simulink model "Lab_3_exerciszcxe"  (R2018a)
settings: Solver=VariableStepAuto  StartTime=0.0  StopTime=7  RelTol=1e-3
libraries: powerlib_extras x7, simulink x3
settings Model: Creator=WIN  LastModifiedBy=WIN

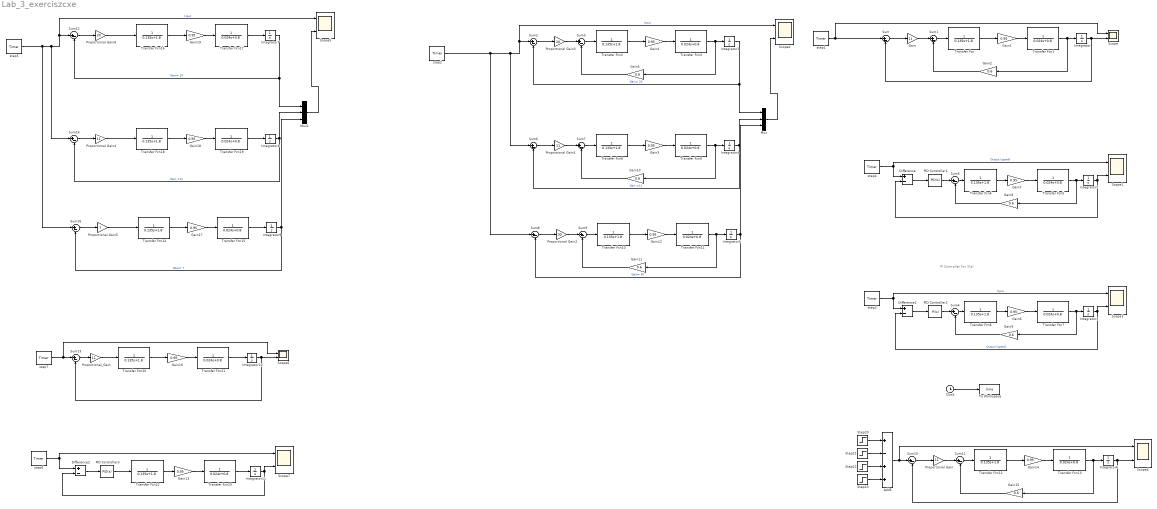
== system Lab_3_exerciszcxe ==
  note: PI Controller For 3(a)
  Add5 : Sum  Inputs=+-++
  Clock : Clock
  Difference : Sum  Inputs=+-
  Difference1 : Sum  Inputs=+-
  Difference2 : Sum  Inputs=+-
  Gain : Gain  Gain=11
  Gain{1,3..4,6..7,12..14,16..19} (12 alike) : Gain  Gain=0.95
  Gain{2,5,8..11,15} (7 alike) : Gain  Gain=0.6
  Integrator{,1..11} (12 alike) : Integrator
  Mux : Mux  Inputs=3
  Mux1 : Mux  Inputs=3
  PID Controller1 : simulink/Continuous/PID Controller  Controller=PID  TimeDomain=Continuous-time  SampleTime=-1  IntegratorMethod=Forward Euler  FilterMethod=Forward Euler  Form=Parallel  UseFilter=on  ControllerParametersSource=internal  P=26  I=12  D=1.5  N=100  InitialConditionSource=internal  InitialConditionForIntegrator=0  InitialConditionForFilter=0  ExternalReset=none  ZeroCross=off  LimitOutput=off  UpperSaturationLimit=inf  LowerSaturationLimit=-inf  LinearizeAsGain=on  AntiWindupMode=none  Kb=1  TrackingMode=off  Kt=1  PParamMin=[]  PParamMax=[]  IParamMin=[]  IParamMax=[]  DParamMin=[]  DParamMax=[]  NParamMin=[]  NParamMax=[]  KbParamMin=[]  KbParamMax=[]  KtParamMin=[]  KtParamMax=[]  POutMin=[]  POutMax=[]  IOutMin=[]  IOutMax=[]  DOutMin=[]  DOutMax=[]  NOutMin=[]  NOutMax=[]  KbOutMin=[]  KbOutMax=[]  KtOutMin=[]  KtOutMax=[]  IntegratorOutMin=[]  IntegratorOutMax=[]  FilterOutMin=[]  FilterOutMax=[]  SumOutMin=[]  SumOutMax=[]  SumI1OutMin=[]  SumI1OutMax=[]  SumI2OutMin=[]  SumI2OutMax=[]  SumI3OutMin=[]  SumI3OutMax=[]  SumDOutMin=[]  SumDOutMax=[]  SaturationOutMin=[]  SaturationOutMax=[]  IntegratorContinuousStateAttributes=''  IntegratorStateMustResolveToSignalObject=off  IntegratorRTWStateStorageClass=Auto  FilterContinuousStateAttributes=''  FilterStateMustResolveToSignalObject=off  FilterRTWStateStorageClass=Auto  DifferentiatorICPrevScaledInput=0  DifferentiatorOutMin=[]  DifferentiatorOutMax=[]  FilterDiffOutCoefMin=[]  FilterDiffOutCoefMax=[]  SumDenOutMin=[]  SumDenOutMax=[]  SumNumOutMin=[]  SumNumOutMax=[]  ReciprocalOutMin=[]  ReciprocalOutMax=[]  DivideOutMin=[]  DivideOutMax=[]  TunerSelectOption=Transfer Function Based (PID Tuner App)
  PID Controller2 : simulink/Continuous/PID Controller  Controller=PI  TimeDomain=Continuous-time  SampleTime=-1  IntegratorMethod=Forward Euler  FilterMethod=Forward Euler  Form=Parallel  UseFilter=on  ControllerParametersSource=internal  P=26  I=12  D=1.5  N=100  InitialConditionSource=internal  InitialConditionForIntegrator=0  InitialConditionForFilter=0  ExternalReset=none  ZeroCross=off  LimitOutput=off  UpperSaturationLimit=inf  LowerSaturationLimit=-inf  LinearizeAsGain=on  AntiWindupMode=none  Kb=1  TrackingMode=off  Kt=1  PParamMin=[]  PParamMax=[]  IParamMin=[]  IParamMax=[]  DParamMin=[]  DParamMax=[]  NParamMin=[]  NParamMax=[]  KbParamMin=[]  KbParamMax=[]  KtParamMin=[]  KtParamMax=[]  POutMin=[]  POutMax=[]  IOutMin=[]  IOutMax=[]  DOutMin=[]  DOutMax=[]  NOutMin=[]  NOutMax=[]  KbOutMin=[]  KbOutMax=[]  KtOutMin=[]  KtOutMax=[]  IntegratorOutMin=[]  IntegratorOutMax=[]  FilterOutMin=[]  FilterOutMax=[]  SumOutMin=[]  SumOutMax=[]  SumI1OutMin=[]  SumI1OutMax=[]  SumI2OutMin=[]  SumI2OutMax=[]  SumI3OutMin=[]  SumI3OutMax=[]  SumDOutMin=[]  SumDOutMax=[]  SaturationOutMin=[]  SaturationOutMax=[]  IntegratorContinuousStateAttributes=''  IntegratorStateMustResolveToSignalObject=off  IntegratorRTWStateStorageClass=Auto  FilterContinuousStateAttributes=''  FilterStateMustResolveToSignalObject=off  FilterRTWStateStorageClass=Auto  DifferentiatorICPrevScaledInput=0  DifferentiatorOutMin=[]  DifferentiatorOutMax=[]  FilterDiffOutCoefMin=[]  FilterDiffOutCoefMax=[]  SumDenOutMin=[]  SumDenOutMax=[]  SumNumOutMin=[]  SumNumOutMax=[]  ReciprocalOutMin=[]  ReciprocalOutMax=[]  DivideOutMin=[]  DivideOutMax=[]  TunerSelectOption=Transfer Function Based (PID Tuner App)
  PID Controller3 : simulink/Continuous/PID Controller  Controller=PID  TimeDomain=Continuous-time  SampleTime=-1  IntegratorMethod=Forward Euler  FilterMethod=Forward Euler  Form=Parallel  UseFilter=on  ControllerParametersSource=internal  P=26  I=12  D=1.5  N=100  InitialConditionSource=internal  InitialConditionForIntegrator=0  InitialConditionForFilter=0  ExternalReset=none  ZeroCross=off  LimitOutput=off  UpperSaturationLimit=inf  LowerSaturationLimit=-inf  LinearizeAsGain=on  AntiWindupMode=none  Kb=1  TrackingMode=off  Kt=1  PParamMin=[]  PParamMax=[]  IParamMin=[]  IParamMax=[]  DParamMin=[]  DParamMax=[]  NParamMin=[]  NParamMax=[]  KbParamMin=[]  KbParamMax=[]  KtParamMin=[]  KtParamMax=[]  POutMin=[]  POutMax=[]  IOutMin=[]  IOutMax=[]  DOutMin=[]  DOutMax=[]  NOutMin=[]  NOutMax=[]  KbOutMin=[]  KbOutMax=[]  KtOutMin=[]  KtOutMax=[]  IntegratorOutMin=[]  IntegratorOutMax=[]  FilterOutMin=[]  FilterOutMax=[]  SumOutMin=[]  SumOutMax=[]  SumI1OutMin=[]  SumI1OutMax=[]  SumI2OutMin=[]  SumI2OutMax=[]  SumI3OutMin=[]  SumI3OutMax=[]  SumDOutMin=[]  SumDOutMax=[]  SaturationOutMin=[]  SaturationOutMax=[]  IntegratorContinuousStateAttributes=''  IntegratorStateMustResolveToSignalObject=off  IntegratorRTWStateStorageClass=Auto  FilterContinuousStateAttributes=''  FilterStateMustResolveToSignalObject=off  FilterRTWStateStorageClass=Auto  DifferentiatorICPrevScaledInput=0  DifferentiatorOutMin=[]  DifferentiatorOutMax=[]  FilterDiffOutCoefMin=[]  FilterDiffOutCoefMax=[]  SumDenOutMin=[]  SumDenOutMax=[]  SumNumOutMin=[]  SumNumOutMax=[]  ReciprocalOutMin=[]  ReciprocalOutMax=[]  DivideOutMin=[]  DivideOutMax=[]  TunerSelectOption=Transfer Function Based (PID Tuner App)
  Proportional Gain : Gain  Gain=11
  Proportional Gain1 : Gain  Gain=11
  Proportional Gain2 : Gain  Gain=30
  Proportional Gain3 : Gain  Gain=20
  Proportional Gain4 : Gain  Gain=11
  Proportional Gain5 : Gain  Gain=7
  Proportional Gain6 : Gain  Gain=20
  Proportional_Gain : Gain  Gain=11
  Scope{,1..7} (8 alike) : Scope  NumInputPorts=2
  Step20 : Step  Time=0  Before=20  After=20  SampleTime=0
  Step21 : Step  Time=5  After=10  SampleTime=0
  Step22 : Step  Time=7  After=20  SampleTime=0
  Step23 : Step  Time=9  After=20  SampleTime=0
  Sum{,1..14,16} (16 alike) : Sum  Inputs=|+-
  To Workspace : ToWorkspace  VariableName=time  SaveFormat=Structure With Time  SampleTime=-1
  Transfer Fcn{,2,4,6,8,10,12,14,16,18,20,22} (12 alike) : TransferFcn  Denominator=[0.135 1.8]
  Transfer Fcn{1,3,5,7,9,11,13,15,17,19,21,23} (12 alike) : TransferFcn  Denominator=[0.024 0.8]
  step1 : powerlib_extras/Control  Blocks/Timer  t=[0 5 7 9]  e=[20 10 30 50]
      settings: SourceProductBaseCode=PS
  step{2..7} (6 alike) : powerlib_extras/Control  Blocks/Timer  t=[0 2 3 5]  e=[20 10 30 50]
      settings: SourceProductBaseCode=PS
  wires:
  Sum/1 -> Gain/1
  Gain/1 -> Sum1/1
  Sum1/1 -> Transfer Fcn/1
  Transfer Fcn/1 -> Gain1/1
  Gain1/1 -> Transfer Fcn1/1
  Transfer Fcn1/1 -> Gain2/1, Integrator/1
  step1/1 -> Scope/1, Sum/1
  Integrator/1 -> Scope/2, Sum/2
  Gain2/1 -> Sum1/2
  Gain5/1 -> Sum3/2
  Integrator1/1 -> Mux/1, Sum2/2  "Gain= 20"
  step2/1 -> Sum8/1, Sum6/1, Scope2/1, Sum2/1  "Input"
  Transfer Fcn3/1 -> Integrator1/1, Gain5/1
  Gain4/1 -> Transfer Fcn3/1
  Transfer Fcn2/1 -> Gain4/1
  Sum3/1 -> Transfer Fcn2/1
  Proportional Gain3/1 -> Sum3/1
  Sum2/1 -> Proportional Gain3/1
  PID Controller1/1 -> Sum5/1
  Sum5/1 -> Transfer Fcn4/1
  Transfer Fcn4/1 -> Gain7/1
  Gain7/1 -> Transfer Fcn5/1
  Transfer Fcn5/1 -> Gain8/1, Integrator2/1
  Integrator2/1 -> Scope1/2, Difference/2
  Gain8/1 -> Sum5/2
  Difference/1 -> PID Controller1/1
  step4/1 -> Scope1/1, Difference/1  "Output (spped)"
  Clock/1 -> To Workspace/1
  step3/1 -> Difference1/1, Scope3/1  "Input"
  Difference1/1 -> PID Controller2/1
  Gain9/1 -> Sum4/2
  Integrator3/1 -> Difference1/2, Scope3/2  "Output (speed)"
  Transfer Fcn7/1 -> Integrator3/1, Gain9/1
  Gain6/1 -> Transfer Fcn7/1
  Transfer Fcn6/1 -> Gain6/1
  Sum4/1 -> Transfer Fcn6/1
  PID Controller2/1 -> Sum4/1
  Sum6/1 -> Proportional Gain1/1
  Proportional Gain1/1 -> Sum7/1
  Sum7/1 -> Transfer Fcn8/1
  Transfer Fcn8/1 -> Gain3/1
  Gain3/1 -> Transfer Fcn9/1
  Transfer Fcn9/1 -> Gain10/1, Integrator4/1
  Integrator4/1 -> Mux/2, Sum6/2  "Gain =11"
  Gain10/1 -> Sum7/2
  Gain11/1 -> Sum9/2
  Integrator5/1 -> Mux/3, Sum8/2  "Gain= 30"
  Transfer Fcn11/1 -> Integrator5/1, Gain11/1
  Gain12/1 -> Transfer Fcn11/1
  Transfer Fcn10/1 -> Gain12/1
  Sum9/1 -> Transfer Fcn10/1
  Proportional Gain2/1 -> Sum9/1
  Sum8/1 -> Proportional Gain2/1
  Mux/1 -> Scope2/2
  Gain15/1 -> Sum11/2
  Integrator6/1 -> Sum10/2, Scope4/2
  Add5/1 -> Sum10/1, Scope4/1
  Transfer Fcn13/1 -> Integrator6/1, Gain15/1
  Gain14/1 -> Transfer Fcn13/1
  Transfer Fcn12/1 -> Gain14/1
  Sum11/1 -> Transfer Fcn12/1
  Proportional Gain/1 -> Sum11/1
  Sum10/1 -> Proportional Gain/1
  Step23/1 -> Add5/4
  Step22/1 -> Add5/3
  Step21/1 -> Add5/2
  Step20/1 -> Add5/1
  Mux1/1 -> Scope5/2
  Sum16/1 -> Proportional Gain5/1
  Proportional Gain5/1 -> Transfer Fcn14/1
  Transfer Fcn14/1 -> Gain17/1
  Gain17/1 -> Transfer Fcn15/1
  Transfer Fcn15/1 -> Integrator9/1
  Integrator9/1 -> Sum16/2, Mux1/3  "Gain= 7"
  Integrator8/1 -> Sum14/2, Mux1/2  "Gain =11"
  Transfer Fcn19/1 -> Integrator8/1
  Gain18/1 -> Transfer Fcn19/1
  Transfer Fcn18/1 -> Gain18/1
  Proportional Gain4/1 -> Transfer Fcn18/1
  Sum14/1 -> Proportional Gain4/1
  Sum12/1 -> Proportional Gain6/1
  Proportional Gain6/1 -> Transfer Fcn16/1
  Transfer Fcn16/1 -> Gain19/1
  Gain19/1 -> Transfer Fcn17/1
  Transfer Fcn17/1 -> Integrator7/1
  step5/1 -> Sum12/1, Scope5/1, Sum14/1, Sum16/1  "Input"
  Integrator7/1 -> Sum12/2, Mux1/1  "Gain= 20"
  Integrator10/1 -> Sum13/2, Scope6/2
  step7/1 -> Sum13/1, Scope6/1
  Transfer Fcn21/1 -> Integrator10/1
  Gain16/1 -> Transfer Fcn21/1
  Transfer Fcn20/1 -> Gain16/1
  Proportional_Gain/1 -> Transfer Fcn20/1
  Sum13/1 -> Proportional_Gain/1
  step6/1 -> Difference2/1, Scope7/1
  Difference2/1 -> PID Controller3/1
  Integrator11/1 -> Difference2/2, Scope7/2
  Transfer Fcn23/1 -> Integrator11/1
  Gain13/1 -> Transfer Fcn23/1
  Transfer Fcn22/1 -> Gain13/1
  PID Controller3/1 -> Transfer Fcn22/1
